simulink model "ps2"  (R2020b)
settings: Solver=VariableStepAuto  StartTime=0.0  StopTime=10  RelTol=1e-3
model workspace (MAT data in the model file):
  M1 = 2500
  M2 = 320
  b = 350
  k1 = 80000
  k2 = 500000
settings Model: Creator=prana  LastModifiedBy=prana

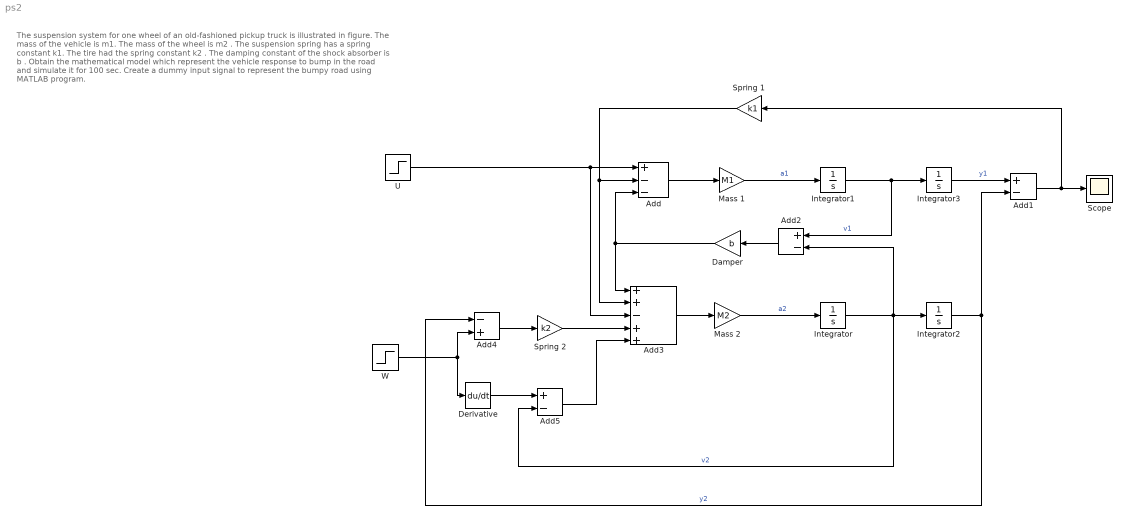
== system ps2 ==
  note: The suspension system for one wheel of an old-fashioned pickup truck is illustrated in figure.
      | The mass of the vehicle is m1.
      | The mass of the wheel is m2 .
      | The suspension spring has a spring constant k1.
      | The tire had the spring constant k2 .
      | The damping constant of the shock absorber is b .
      | Obtain the mathematical model which represent the vehicle response to bump in the road and simulate it for 100 sec. Create a dummy input signal to represent the bumpy road using MATLAB program.
  Add : Sum  Inputs=+--
  Add1 : Sum  Inputs=+-
  Add2 : Sum  Inputs=+-
  Add3 : Sum  Inputs=++-++
  Add4 : Sum  Inputs=-+
  Add5 : Sum  Inputs=+-
  Damper : Gain  Gain=b
  Derivative : Derivative
  Integrator{,1..3} (4 alike) : Integrator
  Mass 1 : Gain  Gain=M1
  Mass 2 : Gain  Gain=M2
  Scope : Scope
  Spring 1 : Gain  Gain=k1
  Spring 2 : Gain  Gain=k2
  U : Step  SampleTime=0
  W : Step  SampleTime=0
  wires:
  U/1 -> Add3/3, Add/1
  Add/1 -> Mass 1/1
  Mass 1/1 -> Integrator1/1  "a1"
  Integrator1/1 -> Add2/1, Integrator3/1  "v1"
  Integrator3/1 -> Add1/1  "y1"
  Integrator/1 -> Add2/2, Integrator2/1, Add5/2  "v2"
  Mass 2/1 -> Integrator/1  "a2"
  Add3/1 -> Mass 2/1
  Add4/1 -> Spring 2/1
  W/1 -> Derivative/1, Add4/2
  Derivative/1 -> Add5/1
  Spring 1/1 -> Add/2, Add3/2
  Spring 2/1 -> Add3/4
  Add1/1 -> Spring 1/1, Scope/1
  Integrator2/1 -> Add1/2, Add4/1  "y2"
  Add2/1 -> Damper/1
  Add5/1 -> Add3/5
  Damper/1 -> Add3/1, Add/3
